simulink model "hpipm_simulink"  (R2017b)
settings: Solver=VariableStepAuto  StartTime=0.0  StopTime=50.0  RelTol=1e-3
undefined symbols (not defined in the file or in its folder): x0
settings Model: Creator=andrea  LastModifiedBy=andrea

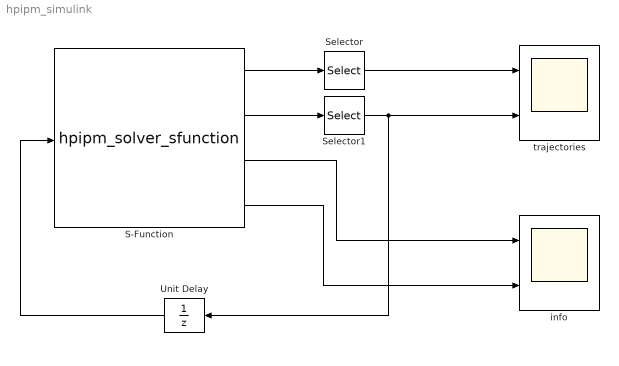
== system hpipm_simulink ==
  S-Function : S-Function  FunctionName=hpipm_solver_sfunction  SFunctionDeploymentMode=off  EnableBusSupport=off
  Selector : Selector  InputPortWidth=90  IndexOptions=Index vector (dialog)  Indices=1:3  OutputSizes=1
  Selector1 : Selector  InputPortWidth=248  IndexOptions=Index vector (dialog)  Indices=9:16  OutputSizes=1
  Unit Delay : UnitDelay  InitialCondition=x0  SampleTime=0.5
  info : Scope  NumInputPorts=2
  trajectories : Scope  NumInputPorts=2
  wires:
  S-Function/2 -> Selector1/1
  Unit Delay/1 -> S-Function/1
  S-Function/1 -> Selector/1
  Selector/1 -> trajectories/1
  Selector1/1 -> Unit Delay/1, trajectories/2
  S-Function/3 -> info/1
  S-Function/4 -> info/2
